simulink model "Ex4_Discrete_Continuous_Sys"  (R2017a)
settings: Solver=VariableStepAuto  StartTime=0.0  StopTime=10  FixedStep=.01  RelTol=1e-3
undefined symbols (not defined in the file or in its folder): b, DiscIntNeverNeededParam, k, m
settings Model: Creator=sulaymon.eshkabilov  LastModifiedBy=sulaymon.eshkabilov

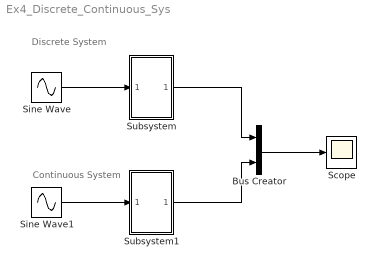
== system Ex4_Discrete_Continuous_Sys ==
  note: Discrete
      | System
  note: Continuous
      | System
  Bus Creator : BusCreator  Inputs=2
  Scope : Scope
  Sine Wave : Sin  Amplitude=2.3  Frequency=131  SampleTime=0.0001
  Sine Wave1 : Sin  Amplitude=2.3  Frequency=131  SampleTime=0
  Subsystem : Subsystem
  Subsystem1 : Subsystem
  wires:
  Bus Creator/1 -> Scope/1
  Sine Wave/1 -> Subsystem/1(In1)
  Subsystem/1(Out1) -> Bus Creator/1
  Sine Wave1/1 -> Subsystem1/1(In1)
  Subsystem1/1(Out1) -> Bus Creator/2

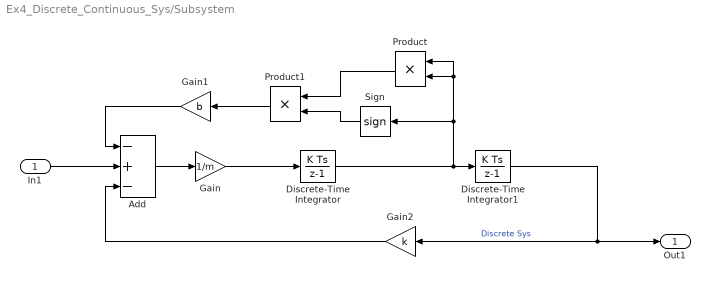
== system Ex4_Discrete_Continuous_Sys/Subsystem ==
  In1 : Inport
  Add : Sum  Inputs=-+-
  Discrete-Time Integrator : DiscreteIntegrator  InitialConditionSetting=State (most efficient)  SampleTime=-1  ICPrevOutput=DiscIntNeverNeededParam  ICPrevScaledInput=DiscIntNeverNeededParam
  Discrete-Time Integrator1 : DiscreteIntegrator  InitialConditionSetting=State (most efficient)  SampleTime=-1  ICPrevOutput=DiscIntNeverNeededParam  ICPrevScaledInput=DiscIntNeverNeededParam
  Gain : Gain  Gain=1/m
  Gain1 : Gain  Gain=b
  Gain2 : Gain  Gain=k
  Product : Product
  Product1 : Product
  Sign : Signum
  Out1 : Outport
  wires:
  In1/1 -> Add/2
  Gain2/1 -> Add/3
  Sign/1 -> Product1/2
  Product/1 -> Product1/1
  Gain1/1 -> Add/1
  Product1/1 -> Gain1/1
  Add/1 -> Gain/1
  Discrete-Time Integrator/1 -> Sign/1, Product/1, Product/2, Discrete-Time Integrator1/1
  Discrete-Time Integrator1/1 -> Out1/1, Gain2/1  "Discrete Sys"
  Gain/1 -> Discrete-Time Integrator/1

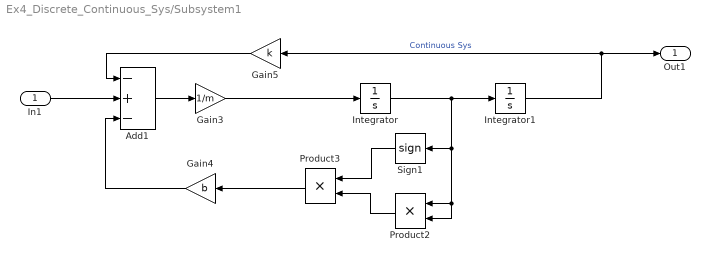
== system Ex4_Discrete_Continuous_Sys/Subsystem1 ==
  In1 : Inport
  Add1 : Sum  Inputs=-+-
  Gain3 : Gain  Gain=1/m
  Gain4 : Gain  Gain=b
  Gain5 : Gain  Gain=k
  Integrator : Integrator
  Integrator1 : Integrator
  Product2 : Product
  Product3 : Product
  Sign1 : Signum
  Out1 : Outport
  wires:
  Add1/1 -> Gain3/1
  In1/1 -> Add1/2
  Gain5/1 -> Add1/1
  Product2/1 -> Product3/2
  Gain3/1 -> Integrator/1
  Sign1/1 -> Product3/1
  Gain4/1 -> Add1/3
  Integrator/1 -> Integrator1/1, Product2/2, Product2/1, Sign1/1
  Integrator1/1 -> Out1/1, Gain5/1  "Continuous Sys"
  Product3/1 -> Gain4/1
